simulink model "h6p3"  (R2024b)
settings: Solver=FixedStepAuto  StartTime=0.0  StopTime=25  FixedStep=.1  RelTol=1e-3
values from neighbouring files (symbols this model uses):
  noise = 1    [h6.m]
  Q = eye(2) * 0.01    [h6.m]
  R = 1    [h6.m]
undefined symbols (not defined in the file or in its folder): A_d, B_d, C_d, D_d
libraries: simulink x2
settings Model: Creator=chrissheehan  LastModifiedBy=chrissheehan

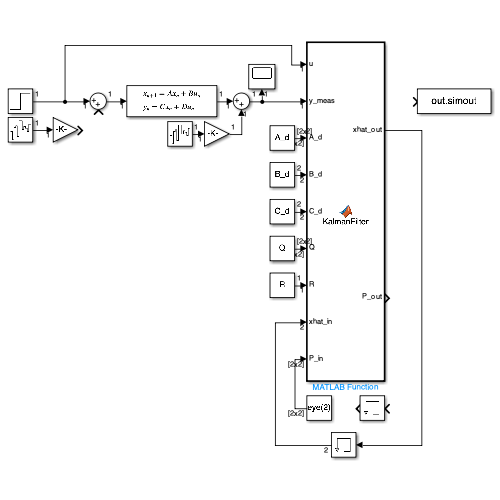
[thumbnail: Simulink's stored preview of the top-level diagram]
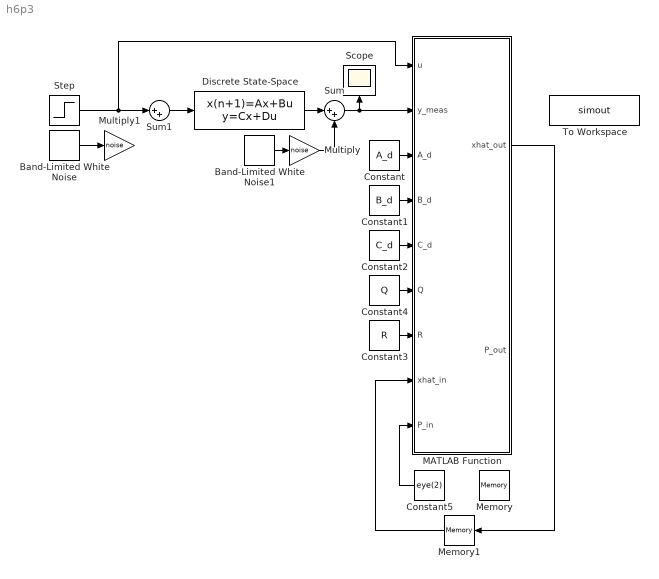
== system h6p3 ==
  Band-Limited White Noise : simulink/Sources/Band-Limited White Noise  Cov=[0.0005]  Ts=0.1  seed=[23341]
  Band-Limited White Noise1 : simulink/Sources/Band-Limited White Noise  Cov=[0.0000005]  Ts=0.1  seed=[23341]
  Constant : Constant  Value=A_d
  Constant1 : Constant  Value=B_d
  Constant2 : Constant  Value=C_d
  Constant3 : Constant  Value=R
  Constant4 : Constant  Value=Q
  Constant5 : Constant  Value=eye(2)
  Discrete State-Space : DiscreteStateSpace  A=A_d  B=B_d  C=C_d  D=D_d  InitialCondition=[0.05, -0.01]  SampleTime=.1
  MATLAB Function : MATLAB Function  TreatAsAtomicUnit=on
  Memory : Memory  InitialCondition=eye(2)
  Memory1 : Memory  InitialCondition=[0; 0]
  Multiply : Gain  Gain=noise
  Multiply1 : Gain  Gain=noise
  Scope : Scope
  Step : Step  Time=0  SampleTime=0
  Sum : Sum  Inputs=|++
  Sum1 : Sum  Inputs=|++
  To Workspace : ToWorkspace  VariableName=simout  SaveFormat=Timeseries  SampleTime=-1
  wires:
  Sum/1 -> MATLAB Function/2(y_meas), Scope/1
  Sum1/1 -> Discrete State-Space/1
  Step/1 -> MATLAB Function/1(u), Sum1/1
  Band-Limited White Noise1/1 -> Multiply/1
  Multiply/1 -> Sum/2
  Band-Limited White Noise/1 -> Multiply1/1
  Discrete State-Space/1 -> Sum/1
  Constant/1 -> MATLAB Function/3(A_d)
  Constant3/1 -> MATLAB Function/7(R)
  Constant4/1 -> MATLAB Function/6(Q)
  Constant2/1 -> MATLAB Function/5(C_d)
  Constant1/1 -> MATLAB Function/4(B_d)
  Memory1/1 -> MATLAB Function/8(xhat_in)
  MATLAB Function/1(xhat_out) -> Memory1/1
  Constant5/1 -> MATLAB Function/9(P_in)

== matlab function h6p3/MATLAB Function ==
  data: u input; xhat_out output; y_meas input; A_d input; B_d input; C_d input; Q input; R input; xhat_in input; P_in input; P_out output
function [xhat_out, P_out] = KalmanFilter(u, y_meas, ...
                                          A_d, B_d, C_d, Q, R, ...
                                          xhat_in, P_in)
% KALMANFILTER  Discrete-time Kalman filter update
%
% Inputs:
%   u        - control input at time k
%   y_meas   - measurement y[k]
%   A_d,B_d,C_d - discrete system matrices
%   Q,R      - process & measurement noise covariances
%   xhat_in  - previous state estimate, xhat[k-1|k-1]
%   P_in     - previous covariance, P[k-1|k-1]
%
% Outputs:
%   xhat_out - updated state estimate, xhat[k|k]
%   P_out    - updated covariance, P[k|k]

% 1) Prediction
xhat_predict = A_d * xhat_in + B_d * u;
P_predict    = A_d * P_in * A_d' + Q;

C_d = [1 0];



% 2) Correction

K = P_predict * C_d' / (C_d * P_predict * C_d' + R);
xhat_out = xhat_predict + K * (y_meas - C_d*xhat_predict);
P_out = (eye(size(A_d)) - K*C_d) * P_predict;
